simulink model "sllookuptable"  (R2020a)
settings: Solver=FixedStepDiscrete  StartTime=0.0  StopTime=12  RelTol=1e-3  EnableMultiTasking=on
PreLoadFcn:
  | Ts = 0.1;
  | Plant = c2d(zpk([],[-1 -3 -5],1),Ts);
  | C0 = pid(1,1,1,'Ts',Ts,'IF','B','DF','B'); % define PID structure
  | C = pidtune(Plant,C0); % design PID
  | [Kp Ki Kd] = piddata(C); % obtain PID gains
  | FIS = sugfis;
  | FIS = addInput(FIS,[-10 10],'Name','E');
  | FIS = addMF(FIS,'E','gaussmf',[7 -10],'Name','Negative');
  | FIS = addMF(FIS,'E','gaussmf',[7 10],'Name','Positive');
  | FIS = addInput(FIS,[-10 10],'Name','CE');
  | FIS = addMF(FIS,'CE','gaussmf',[7 -10],'Name','Negative');
  | FIS = addMF(FIS,'CE','gaussmf',[7 10],'Name','Positive');
  | FIS = addOutput(FIS,[-20 20],'Name','u');
  | FIS = addMF(FIS,'u','constant',-20,'Name','Min');
  | FIS = addMF(FIS,'u','constant',0,'Name','Zero');
  | FIS = addMF(FIS,'u','constant',20,'Name','Max');
  | ruleList = [1 1 1 1 1;...   % Rule 1
  |             1 2 2 1 1;...   % Rule 2
  |             2 1 2 1 1;...   % Rule 3
  |             2 2 3 1 1];     % Rule 4
  | FIS = addRule(FIS,ruleList);GE = 10;
  | GCE = GE*(Kp-sqrt(Kp^2-4*Ki*Kd))/2/Ki;
  | GCU = Ki/GE;
  | GU = Kd/GCE;
  | Step = 1; % use 21 break points for both E and CE inputs
  | E = -10:Step:10;
  | CE = -10:Step:10;
  | N = length(E);
  | LookUpTableData = zeros(N);
  | for i=1:N
  |    for j=1:N
  |       % compute output u for each combination of break points
  |       LookUpTableData(i,j) = evalfis(FIS,[E(i) CE(j)]);
  |    end
  | end
undefined symbols (not defined in the file or in its folder): DiscIntNeverNeededParam, Kd, Ki, Kp
libraries: simulink x3, cstblocks x3, fuzblock x1
CloseFcn:
  | clear C E GCU Kd LookUpTableData Step j C0 FIS GE Ki N Ts ruleList CE GCE GU Kp Plant i
settings Model: FPTRunName=Active  Creator=The MathWorks, Inc.  LastModifiedBy=kekatos
settings DataIOCC: LimitDataPoints=on  SaveFormat=Array  ReturnWorkspaceOutputs=off
settings OptimizationCC: ExpressionDepthLimit=2147483647  LifeSpan=inf
settings DebuggingCC: UnderspecifiedInitializationDetection=Classic  MergeDetectMultiDrivingBlocksExec=none  SolverPrmCheckMsg=warning  FcnCallInpInsideContextMsg=warning  StateNameClashWarn=warning  SFUnexpectedBacktrackingDiag=warning  SFNoUnconditionalDefaultTransitionDiag=warning  SFExecutionAtInitializationDiag=none  ArithmeticOperatorsInVariantConditions=warning
settings HardwareCC: ProdBitPerPointer=32  ProdBitPerSizeT=32  ProdBitPerPtrDiffT=32  ProdLargestAtomicFloat=None  ProdIntDivRoundTo=Undefined  ProdEndianess=Unspecified  ProdWordSize=32  ProdHWDeviceType=32-bit Generic
settings ModelReferenceCC: PropagateSignalLabelsOutOfModel=off
settings SFSimCC: SimUseLocalCustomCode=off  CustomCodeUndefinedFunction=UseInterfaceOnly
settings RTWCC: RTWUseLocalCustomCode=off
settings CodeAppCC: StateflowObjectComments=on
settings GRTTargetCC: TargetLangStandard=C89/C90 (ANSI)  CombineOutputUpdateFcns=off  GRTInterface=on
settings ConfigComp: CovMetricSettings=dw  CovHtmlReporting=on  CovSaveCumulativeToWorkspaceVar=on  CovSaveSingleToWorkspaceVar=on  CovExternalEMLEnable=off

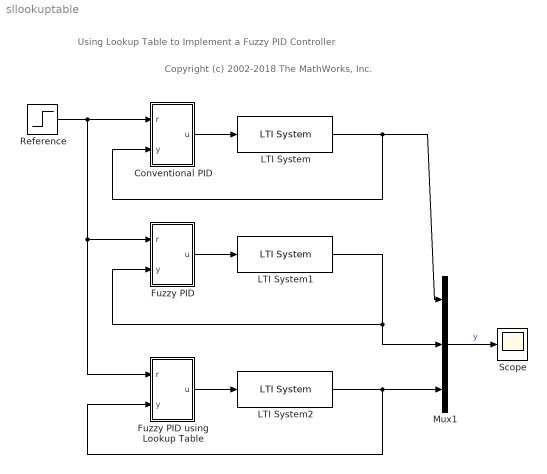
== system sllookuptable ==
  note: Using Lookup Table to Implement a Fuzzy PID Controller
  note: Copyright (c) 2002-2018 The MathWorks, Inc.
  Conventional PID : Subsystem
  Fuzzy PID : Subsystem
  Fuzzy PID using Lookup Table : Subsystem
  LTI System : cstblocks/LTI System  sys=Plant  IC=[]
  LTI System1 : cstblocks/LTI System  sys=Plant  IC=[]
  LTI System2 : cstblocks/LTI System  sys=Plant  IC=[]
  Mux1 : Mux  Inputs=3
  Reference : Step  SampleTime=0
  Scope : Scope
  wires:
  LTI System/1 -> Conventional PID/2(y), Mux1/1
  Conventional PID/1(u) -> LTI System/1
  Reference/1 -> Fuzzy PID/1(r), Fuzzy PID using Lookup Table/1(r), Conventional PID/1(r)
  LTI System1/1 -> Fuzzy PID/2(y), Mux1/2
  Fuzzy PID/1(u) -> LTI System1/1
  LTI System2/1 -> Mux1/3, Fuzzy PID using Lookup Table/2(y)
  Fuzzy PID using Lookup Table/1(u) -> LTI System2/1
  Mux1/1 -> Scope/1  "y"

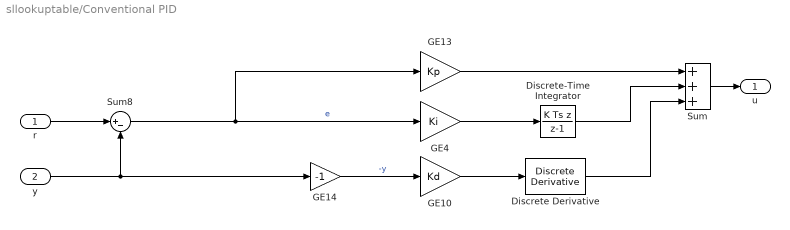
== system sllookuptable/Conventional PID ==
  r : Inport
  y : Inport  Port=2
  Discrete Derivative : simulink/Discrete/Discrete Derivative  gainval=1  ICPrevScaledInput=0.0  OutMin=[]  OutMax=[]  OutDataType=fixdt(1, 16)  OutScaling=2^-10  DoSatur=off
  Discrete-Time Integrator : DiscreteIntegrator  IntegratorMethod=Integration: Backward Euler  gainval=1  SampleTime=Ts  ICPrevOutput=DiscIntNeverNeededParam  ICPrevScaledInput=DiscIntNeverNeededParam
  GE10 : Gain  Gain=Kd
  GE13 : Gain  Gain=Kp
  GE14 : Gain  Gain=-1
  GE4 : Gain  Gain=Ki
  Sum : Sum  Inputs=+++
  Sum8 : Sum  Inputs=|+-
  u : Outport  VectorParamsAs1DForOutWhenUnconnected=off
  wires:
  GE13/1 -> Sum/1
  Sum8/1 -> GE4/1, GE13/1  "e"
  Discrete-Time Integrator/1 -> Sum/2
  GE4/1 -> Discrete-Time Integrator/1
  GE10/1 -> Discrete Derivative/1
  Discrete Derivative/1 -> Sum/3
  GE14/1 -> GE10/1  "-y"
  r/1 -> Sum8/1
  y/1 -> Sum8/2, GE14/1
  Sum/1 -> u/1

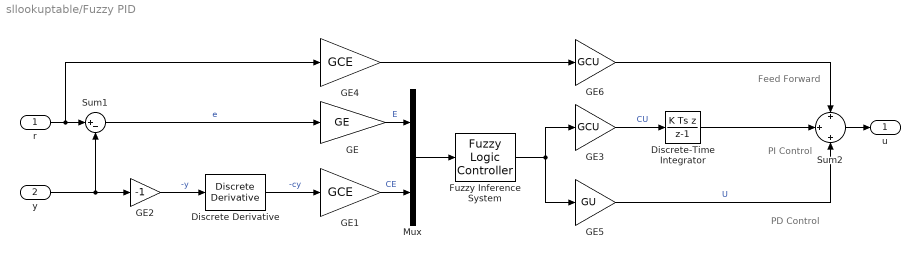
== system sllookuptable/Fuzzy PID ==
  note: PD Control
  note: PI Control
  note: Feed Forward
  r : Inport
  y : Inport  Port=2
  Discrete Derivative : simulink/Discrete/Discrete Derivative  gainval=1  ICPrevScaledInput=0.0  OutMin=[]  OutMax=[]  OutDataType=fixdt(1, 16)  OutScaling=2^-10  DoSatur=off
  Discrete-Time Integrator : DiscreteIntegrator  IntegratorMethod=Integration: Backward Euler  SampleTime=Ts  ICPrevOutput=DiscIntNeverNeededParam  ICPrevScaledInput=DiscIntNeverNeededParam
  Fuzzy Inference System : fuzblock/Fuzzy Logic  Controller  FIS=FIS  OutputSampleNumber=101  DataType=double  FuzzifiedInputs=off  RuleFiringStrengths=off  RuleOutputs=off  AggregatedOutputs=off  SimulateUsing=Interpreted execution  OutOfRangeInputValueMessage=warning  NoRuleFiredMessage=warning  EmptyOutputFuzzySetMessage=warning
  GE : Gain  Gain=GE
  GE1 : Gain  Gain=GCE
  GE2 : Gain  Gain=-1
  GE3 : Gain  Gain=GCU
  GE4 : Gain  Gain=GCE
  GE5 : Gain  Gain=GU
  GE6 : Gain  Gain=GCU
  Mux : Mux  Inputs=2
  Sum1 : Sum  Inputs=|+-
  Sum2 : Sum  Inputs=+|+|+
  u : Outport  VectorParamsAs1DForOutWhenUnconnected=off
  wires:
  Sum1/1 -> GE/1  "e"
  Mux/1 -> Fuzzy Inference System/1
  GE/1 -> Mux/1  "E"
  GE1/1 -> Mux/2  "CE"
  Fuzzy Inference System/1 -> GE3/1, GE5/1
  GE3/1 -> Discrete-Time Integrator/1  "CU"
  GE5/1 -> Sum2/3  "U"
  GE2/1 -> Discrete Derivative/1  "-y"
  Discrete Derivative/1 -> GE1/1  "-cy"
  r/1 -> Sum1/1, GE4/1
  y/1 -> Sum1/2, GE2/1
  Sum2/1 -> u/1
  GE4/1 -> GE6/1
  Discrete-Time Integrator/1 -> Sum2/2
  GE6/1 -> Sum2/1

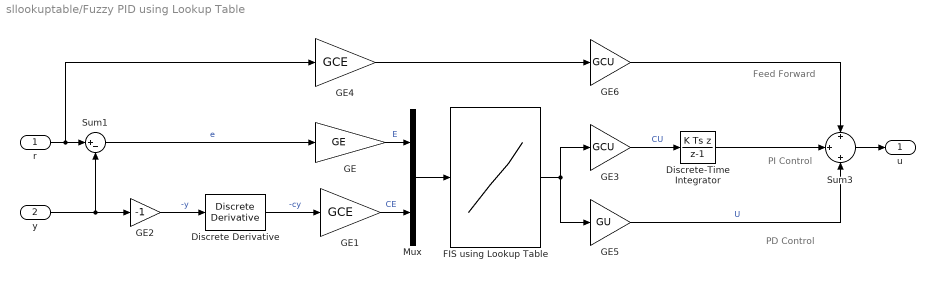
== system sllookuptable/Fuzzy PID using Lookup Table ==
  note: PI Control
  note: PD Control
  note: Feed Forward
  r : Inport
  y : Inport  Port=2
  Discrete Derivative : simulink/Discrete/Discrete Derivative  gainval=1  ICPrevScaledInput=0.0  OutMin=[]  OutMax=[]  OutDataType=fixdt(1, 16)  OutScaling=2^-10  DoSatur=off
  Discrete-Time Integrator : DiscreteIntegrator  IntegratorMethod=Integration: Backward Euler  SampleTime=Ts  ICPrevOutput=DiscIntNeverNeededParam  ICPrevScaledInput=DiscIntNeverNeededParam
  FIS using Lookup Table : Lookup_n-D  BreakpointsForDimension1=E  BreakpointsForDimension2=CE  UseOneInputPortForAllInputData=on  Table=LookUpTableData  RndMeth=Simplest  InputSameDT=on
  GE : Gain  Gain=GE
  GE1 : Gain  Gain=GCE
  GE2 : Gain  Gain=-1
  GE3 : Gain  Gain=GCU
  GE4 : Gain  Gain=GCE
  GE5 : Gain  Gain=GU
  GE6 : Gain  Gain=GCU
  Mux : Mux  Inputs=2
  Sum1 : Sum  Inputs=|+-
  Sum3 : Sum  Inputs=+|+|+
  u : Outport  VectorParamsAs1DForOutWhenUnconnected=off
  wires:
  Sum1/1 -> GE/1  "e"
  Mux/1 -> FIS using Lookup Table/1
  GE/1 -> Mux/1  "E"
  GE1/1 -> Mux/2  "CE"
  FIS using Lookup Table/1 -> GE5/1, GE3/1
  GE3/1 -> Discrete-Time Integrator/1  "CU"
  GE5/1 -> Sum3/3  "U"
  GE2/1 -> Discrete Derivative/1  "-y"
  Discrete Derivative/1 -> GE1/1  "-cy"
  r/1 -> Sum1/1, GE4/1
  y/1 -> GE2/1, Sum1/2
  Discrete-Time Integrator/1 -> Sum3/2
  Sum3/1 -> u/1
  GE4/1 -> GE6/1
  GE6/1 -> Sum3/1
